simulink model "gm_sampleModel2016_3_sub"  (R2023a)
settings: Solver=VariableStepAuto  StartTime=0.0  StopTime=10.0  RelTol=1e-3
libraries: simulink x2
settings Model: Creator=user1  LastModifiedBy=user1
settings OptimizationCC: BlockReduction=off  ConditionallyExecuteInputs=off
settings DebuggingCC: InheritedTsInSrcMsg=none

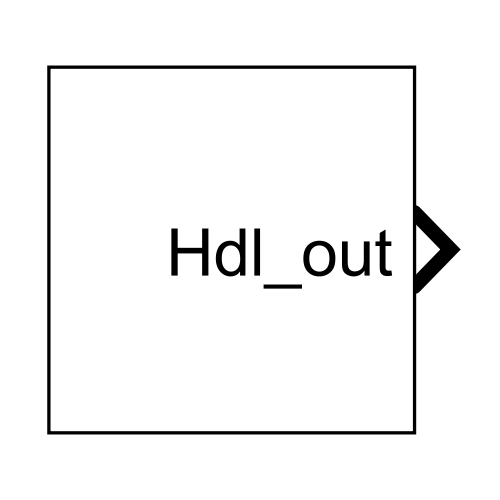
[thumbnail: Simulink's stored preview of the top-level diagram]
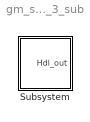
== system gm_sampleModel2016_3_sub ==
  Subsystem : Subsystem

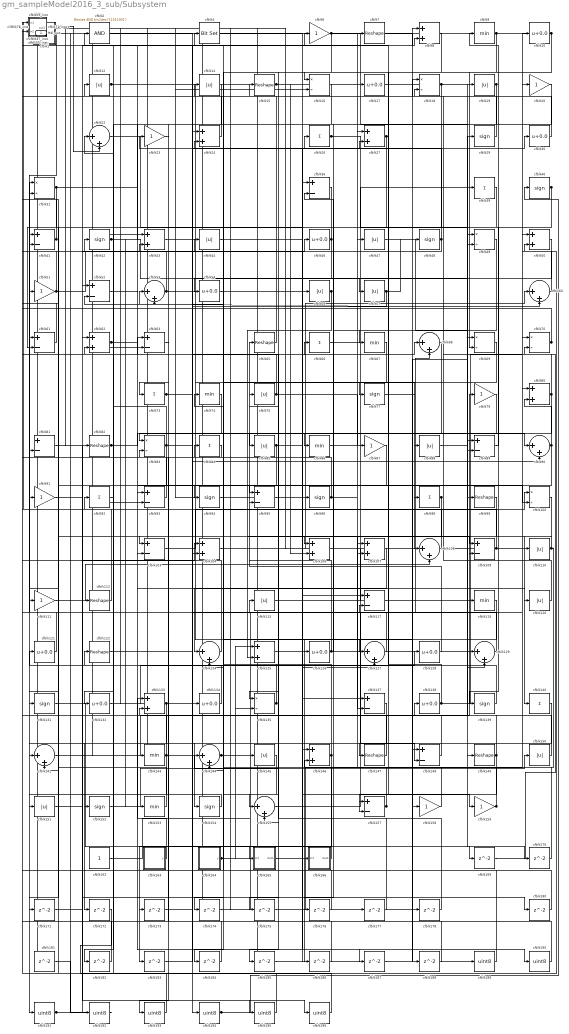
== system gm_sampleModel2016_3_sub/Subsystem ==
  cfblk1 : Subsystem  mask(Compare To Zero){relop=<=, OutDataTypeStr=uint8, ZeroCross=on}
      mask prompts: relop "Simulink:masks:Operator_MP"; OutDataTypeStr "Simulink:masks:OutputDataType_MP"; ZeroCross "Simulink:masks:EnableZerocrossingDetection_MP"
      mask help: Simulink:masks:CompareToZero_MD
      mask init:
      | OutDataTypeStr = 'uint8';
      | ZeroCross = 'on';
      | blkName = 'sampleModel2016_3_sub/Subsystem/cfblk1';
      | relop = '<=';
      | setValue = 'fixdt(0, 8)';
      mask TypeOptions relop: == | ~= | < | <= | >= | >
      mask TypeOptions OutDataTypeStr: Simulink:masks:uint8 | Simulink:masks:boolean
      mask Callback ZeroCross: sl('zeroCrossEnable', gcbh);
      mask Display: disp([relop,' 0'])
  cfblk{10,17,30,46,54,121,126,128,132,134,138} (11 alike) : Bias  Bias=0.0  SaturateOnIntegerOverflow=off
  cfblk{16,18,31,49,69..70,83,100,135} (9 alike) : Product  Inputs=*/  OutDataTypeStr=uint8  RndMeth=Zero  SaturateOnIntegerOverflow=on
  cfblk{36,41,52,61,63,81,89,93,95,103,109,117,137,148,157} (15 alike) : Sum  Inputs=+-  OutDataTypeStr=uint8
  cfblk{8,24,27,43,50,62,80,104,106..107,125,133,146} (13 alike) : Sum  OutDataTypeStr=uint8
  cfblk{22,53,60,68,90,108,124,127,129,141,144,155} (12 alike) : Sum  Inputs=|++  OutDataTypeStr=uint8
  cfblk{12,14,19,44,47,56..57,75,85,88,110,115,120,145,150..151} (16 alike) : Abs  OutDataTypeStr=uint8  SaturateOnIntegerOverflow=off
  cfblk{6,20,23,51,79,87,91,111,158..159} (10 alike) : Gain  OutDataTypeStr=uint8
  cfblk{7,15,65,82,99,112,122,147,149} (9 alike) : Reshape
  cfblk113_inst : Subsystem
  cfblk{9,67,74,86,119,143,153} (7 alike) : MinMax  OutDataTypeStr=uint8
  cfblk123_inst : Subsystem
  cfblk130_inst : Subsystem
  cfblk{29,40,42,48,77,94,96,131,139,152,154} (11 alike) : Signum
  cfblk13_inst : Subsystem
  cfblk{26,39,66,73,84,92,98,140} (8 alike) : Sum  Inputs=+  OutDataTypeStr=uint8
  cfblk156_inst : Subsystem
  cfblk162 : Constant  OutDataTypeStr=uint8  SampleTime=-1
  cfblk163 : Subsystem  mask(Counter Free-Running){NumBits=double(16), tsamp=double(-1)}
      mask prompts: NumBits "Simulink:masks:NumberOfBits_MP"; tsamp "Simulink:masks:SampleTime_MP"
      mask help: Simulink:masks:CounterFreeRunning_MD
  cfblk164 : Subsystem  mask(Counter Limited){uplimit=double(7), tsamp=double(-1)}
      mask prompts: uplimit "Simulink:masks:UpperLimit_MP"; tsamp "Simulink:masks:SampleTime_MP"
      mask help: Simulink:masks:CounterLimited_MD
      mask init:
      | nbits = double(8);
      | tsamp = double(-1);
      | uplimit = double(7);
  cfblk165 : Subsystem
  cfblk166 : Subsystem
  cfblk{169..178,180..188} (19 alike) : Delay  SampleTime=1
  cfblk{189..196} (8 alike) : DataTypeConversion  OutDataTypeStr=uint8  SaturateOnIntegerOverflow=off  RndMeth=Floor
  cfblk2 : simulink/Logic and Bit Operations/Bitwise Operator  logicop=AND  UseBitMask=on  BitMask=bin2dec('11011001')  BitMaskRealWorld=Stored Integer
      settings: LibrarySourceBlock=|
      | hdlsllib/Logic and Bit
      | Operations/Bitwise
      | Operator
  cfblk25_inst : Subsystem
  cfblk3 : Constant  Value=0  OutDataTypeStr=uint8  SampleTime=1
  cfblk37_inst : Subsystem
  cfblk4 : simulink/Logic and Bit Operations/Bit Set  iBit=0
      settings: LibrarySourceBlock=|
      | hdlsllib/Logic and Bit
      | Operations/Bit Set
  cfblk55_inst : Subsystem
  cfblk59_inst : Subsystem
  cfblk71_inst : Subsystem
  cfblk78_inst : Subsystem
  Hdl_out : Outport  OutDataTypeStr=uint8  SampleTime=1
  wires:
  cfblk1/1(y) -> cfblk191/1
  cfblk10/1 -> cfblk69/2, Hdl_out/1
  cfblk100/1 -> cfblk140/1
  cfblk103/1 -> cfblk100/1
  cfblk104/1 -> cfblk60/1
  cfblk106/1 -> cfblk148/2
  cfblk107/1 -> cfblk124/1
  cfblk108/1 -> cfblk37_inst/1(in1)
  cfblk109/1 -> cfblk78_inst/2(in2), cfblk31/1
  cfblk110/1 -> cfblk133/2, cfblk106/1
  cfblk111/1 -> cfblk108/2
  cfblk112/1 -> cfblk13_inst/1(in1)
  cfblk113_inst/1(out1) -> cfblk43/1
  cfblk115/1 -> cfblk39/1
  cfblk117/1 -> cfblk10/1
  cfblk119/1 -> cfblk184/1
  cfblk12/1 -> cfblk90/1, cfblk188/1
  cfblk120/1 -> cfblk18/2
  cfblk121/1 -> cfblk78_inst/1(in1)
  cfblk122/1 -> cfblk66/1
  cfblk123_inst/1(out1) -> cfblk19/1, cfblk134/1, cfblk16/2
  cfblk124/1 -> cfblk123_inst/1(in1)
  cfblk125/1 -> cfblk186/1
  cfblk126/1 -> cfblk65/1, cfblk36/2
  cfblk127/1 -> cfblk115/1
  cfblk128/1 -> cfblk95/2
  cfblk129/1 -> cfblk61/1
  cfblk13_inst/1(out1) -> cfblk189/1
  cfblk130_inst/1(out1) -> cfblk110/1
  cfblk131/1 -> cfblk169/1
  cfblk132/1 -> cfblk128/1
  cfblk133/1 -> cfblk68/1, cfblk141/2
  cfblk134/1 -> cfblk121/1
  cfblk135/1 -> cfblk52/2, cfblk84/1
  cfblk137/1 -> cfblk172/1
  cfblk138/1 -> cfblk130_inst/2(in2), cfblk20/1
  cfblk139/1 -> cfblk122/1
  cfblk14/1 -> cfblk182/1
  cfblk140/1 -> cfblk154/1
  cfblk141/1 -> cfblk49/2
  cfblk143/1 -> cfblk55_inst/2(in2), cfblk151/1
  cfblk144/1 -> cfblk70/1, cfblk135/2
  cfblk145/1 -> cfblk174/1
  cfblk146/1 -> cfblk24/2, cfblk183/1
  cfblk147/1 -> cfblk74/1
  cfblk148/1 -> cfblk75/1
  cfblk149/1 -> cfblk157/2, cfblk79/1
  cfblk15/1 -> cfblk146/1, cfblk117/1, cfblk106/2
  cfblk150/1 -> cfblk12/1
  cfblk151/1 -> cfblk112/1
  cfblk152/1 -> cfblk150/1
  cfblk153/1 -> cfblk51/1
  cfblk154/1 -> cfblk152/1
  cfblk155/1 -> cfblk68/2
  cfblk156_inst/1(out1) -> cfblk63/2, cfblk143/1
  cfblk157/1 -> cfblk62/2, cfblk53/1
  cfblk158/1 -> cfblk92/1
  cfblk159/1 -> cfblk146/2, cfblk14/1
  cfblk16/1 -> cfblk103/1
  cfblk162/1 -> cfblk109/2
  cfblk163/1(y) -> cfblk133/1
  cfblk164/1(y) -> cfblk138/1, cfblk125/1
  cfblk165/1(Out1) -> cfblk47/1
  cfblk166/1(Out1) -> cfblk36/1
  cfblk169/1 -> cfblk70/2
  cfblk17/1 -> cfblk157/1
  cfblk170/1 -> cfblk124/2
  cfblk171/1 -> cfblk104/1
  cfblk172/1 -> cfblk50/2
  cfblk173/1 -> cfblk60/2
  cfblk174/1 -> cfblk107/1
  cfblk175/1 -> cfblk80/1
  cfblk176/1 -> cfblk156_inst/2(in2)
  cfblk177/1 -> cfblk144/1
  cfblk178/1 -> cfblk63/1
  cfblk18/1 -> cfblk131/1, cfblk170/1
  cfblk180/1 -> cfblk25_inst/2(in2)
  cfblk181/1 -> cfblk192/1
  cfblk182/1 -> cfblk123_inst/2(in2)
  cfblk183/1 -> cfblk117/2
  cfblk184/1 -> cfblk71_inst/2(in2)
  cfblk185/1 -> cfblk127/2
  cfblk186/1 -> cfblk24/1
  cfblk187/1 -> cfblk69/1
  cfblk188/1 -> cfblk83/2
  cfblk189/1 -> cfblk4/1
  cfblk19/1 -> cfblk135/1, cfblk86/1
  cfblk190/1 -> cfblk148/1
  cfblk191/1 -> cfblk46/1, cfblk6/1
  cfblk192/1 -> cfblk1/1(u)
  cfblk193/1 -> cfblk2/1
  cfblk194/1 -> cfblk40/1, cfblk196/1
  cfblk195/1 -> cfblk130_inst/1(in1)
  cfblk196/1 -> cfblk91/1
  cfblk2/1 -> cfblk194/1
  cfblk20/1 -> cfblk103/2
  cfblk22/1 -> cfblk166/1(In1)
  cfblk23/1 -> cfblk73/1
  cfblk24/1 -> cfblk71_inst/1(in1)
  cfblk25_inst/1(out1) -> cfblk96/1, cfblk82/1
  cfblk26/1 -> cfblk89/1, cfblk129/2
  cfblk27/1 -> cfblk61/2, cfblk57/1
  cfblk29/1 -> cfblk59_inst/1(in1)
  cfblk3/1 -> cfblk22/2, cfblk181/1
  cfblk30/1 -> cfblk18/1
  cfblk31/1 -> cfblk93/1, cfblk41/2
  cfblk36/1 -> cfblk85/1
  cfblk37_inst/1(out1) -> cfblk56/1
  cfblk39/1 -> cfblk147/1
  cfblk4/1 -> cfblk190/1
  cfblk40/1 -> cfblk155/2, cfblk139/1
  cfblk41/1 -> cfblk55_inst/1(in1), cfblk113_inst/2(in2)
  cfblk42/1 -> cfblk99/1, cfblk8/2, cfblk153/1
  cfblk43/1 -> cfblk77/1
  cfblk44/1 -> cfblk27/2
  cfblk46/1 -> cfblk41/1, cfblk165/1(In1)
  cfblk47/1 -> cfblk149/1
  cfblk48/1 -> cfblk43/2, cfblk23/1
  cfblk49/1 -> cfblk176/1
  cfblk50/1 -> cfblk144/2
  cfblk51/1 -> cfblk44/1, cfblk37_inst/2(in2)
  cfblk52/1 -> cfblk187/1
  cfblk53/1 -> cfblk59_inst/2(in2), cfblk108/1
  cfblk54/1 -> cfblk137/1
  cfblk55_inst/1(out1) -> cfblk81/1, cfblk145/1
  cfblk56/1 -> cfblk125/2, cfblk185/1
  cfblk57/1 -> cfblk53/2, cfblk48/1
  cfblk59_inst/1(out1) -> cfblk178/1, cfblk177/1
  cfblk6/1 -> cfblk89/2, cfblk16/1
  cfblk60/1 -> cfblk50/1
  cfblk61/1 -> cfblk25_inst/1(in1)
  cfblk62/1 -> cfblk120/1, cfblk180/1
  cfblk63/1 -> cfblk193/1
  cfblk65/1 -> cfblk15/1
  cfblk66/1 -> cfblk29/1
  cfblk67/1 -> cfblk126/1
  cfblk68/1 -> cfblk175/1
  cfblk69/1 -> cfblk94/1
  cfblk7/1 -> cfblk158/1
  cfblk70/1 -> cfblk156_inst/1(in1), cfblk31/2
  cfblk71_inst/1(out1) -> cfblk93/2, cfblk17/1, cfblk119/1
  cfblk73/1 -> cfblk8/1, cfblk26/1
  cfblk74/1 -> cfblk83/1
  cfblk75/1 -> cfblk113_inst/1(in1), cfblk87/1
  cfblk77/1 -> cfblk98/1
  cfblk78_inst/1(out1) -> cfblk129/1
  cfblk79/1 -> cfblk127/1
  cfblk8/1 -> cfblk54/1
  cfblk80/1 -> cfblk52/1, cfblk104/2
  cfblk81/1 -> cfblk173/1
  cfblk82/1 -> cfblk88/1, cfblk100/2
  cfblk83/1 -> cfblk90/2, cfblk42/1, cfblk132/1
  cfblk84/1 -> cfblk81/2
  cfblk85/1 -> cfblk141/1, cfblk159/1
  cfblk86/1 -> cfblk27/1
  cfblk87/1 -> cfblk95/1
  cfblk88/1 -> cfblk49/1
  cfblk89/1 -> cfblk9/1
  cfblk9/1 -> cfblk155/1, cfblk67/1
  cfblk90/1 -> cfblk80/2, cfblk111/1
  cfblk91/1 -> cfblk195/1
  cfblk92/1 -> cfblk22/1
  cfblk93/1 -> cfblk62/1
  cfblk94/1 -> cfblk109/1
  cfblk95/1 -> cfblk30/1
  cfblk96/1 -> cfblk7/1, cfblk13_inst/2(in2)
  cfblk98/1 -> cfblk137/2, cfblk171/1
  cfblk99/1 -> cfblk107/2

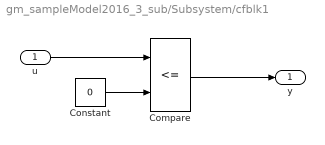
== system gm_sampleModel2016_3_sub/Subsystem/cfblk1 ==
  u : Inport  OutDataTypeStr=uint8  SampleTime=1
  Compare : RelationalOperator  Operator=<=  OutDataTypeStr=fixdt(0, 8)
  Constant : Constant  DisableCoverage=on  Value=0  OutDataTypeStr=Inherit: Inherit via back propagation  SampleTime=-1  PreserveConstantTs=on
  y : Outport  SampleTime=1
  wires:
  u/1 -> Compare/1
  Compare/1 -> y/1
  Constant/1 -> Compare/2

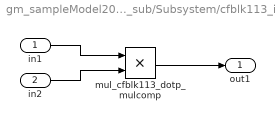
== system gm_sampleModel2016_3_sub/Subsystem/cfblk113_inst ==
  in1 : Inport  OutDataTypeStr=uint8  SampleTime=1
  in2 : Inport  Port=2  OutDataTypeStr=uint8  SampleTime=1
  mul_cfblk113_dotp_mulcomp : Product  Inputs=**  OutDataTypeStr=uint8  SampleTime=1
  out1 : Outport  OutDataTypeStr=uint8  SampleTime=1
  wires:
  in1/1 -> mul_cfblk113_dotp_mulcomp/1
  in2/1 -> mul_cfblk113_dotp_mulcomp/2
  mul_cfblk113_dotp_mulcomp/1 -> out1/1

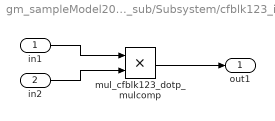
== system gm_sampleModel2016_3_sub/Subsystem/cfblk123_inst ==
  in1 : Inport  OutDataTypeStr=uint8  SampleTime=1
  in2 : Inport  Port=2  OutDataTypeStr=uint8  SampleTime=1
  mul_cfblk123_dotp_mulcomp : Product  Inputs=**  OutDataTypeStr=uint8  SampleTime=1
  out1 : Outport  OutDataTypeStr=uint8  SampleTime=1
  wires:
  in1/1 -> mul_cfblk123_dotp_mulcomp/1
  in2/1 -> mul_cfblk123_dotp_mulcomp/2
  mul_cfblk123_dotp_mulcomp/1 -> out1/1

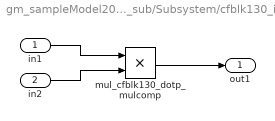
== system gm_sampleModel2016_3_sub/Subsystem/cfblk130_inst ==
  in1 : Inport  OutDataTypeStr=uint8  SampleTime=1
  in2 : Inport  Port=2  OutDataTypeStr=uint8  SampleTime=1
  mul_cfblk130_dotp_mulcomp : Product  Inputs=**  OutDataTypeStr=uint8  SampleTime=1
  out1 : Outport  OutDataTypeStr=uint8  SampleTime=1
  wires:
  in1/1 -> mul_cfblk130_dotp_mulcomp/1
  in2/1 -> mul_cfblk130_dotp_mulcomp/2
  mul_cfblk130_dotp_mulcomp/1 -> out1/1

== system gm_sampleModel2016_3_sub/Subsystem/cfblk13_inst ==
  in1 : Inport  OutDataTypeStr=uint8  SampleTime=1
  in2 : Inport  Port=2  OutDataTypeStr=uint8  SampleTime=1
  mul_cfblk13_dotp_mulcomp : Product  Inputs=**  OutDataTypeStr=uint8  SampleTime=1
  out1 : Outport  OutDataTypeStr=uint8  SampleTime=1
  wires:
  in1/1 -> mul_cfblk13_dotp_mulcomp/1
  in2/1 -> mul_cfblk13_dotp_mulcomp/2
  mul_cfblk13_dotp_mulcomp/1 -> out1/1

== system gm_sampleModel2016_3_sub/Subsystem/cfblk156_inst ==
  in1 : Inport  OutDataTypeStr=uint8  SampleTime=1
  in2 : Inport  Port=2  OutDataTypeStr=uint8  SampleTime=1
  mul_cfblk156_dotp_mulcomp : Product  Inputs=**  OutDataTypeStr=uint8  SampleTime=1
  out1 : Outport  OutDataTypeStr=uint8  SampleTime=1
  wires:
  in1/1 -> mul_cfblk156_dotp_mulcomp/1
  in2/1 -> mul_cfblk156_dotp_mulcomp/2
  mul_cfblk156_dotp_mulcomp/1 -> out1/1

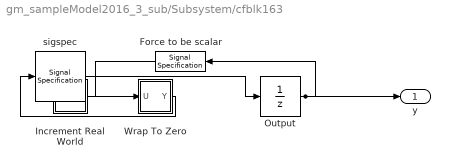
== system gm_sampleModel2016_3_sub/Subsystem/cfblk163 ==
  Force to be scalar : SignalSpecification  DisableCoverage=on  Dimensions=1
  Increment Real World : Subsystem  mask(Real World Value Increment){}
      mask help: Simulink:masks:RealWorldValueIncrement_MD
      mask Display: disp('V++')
  Output : UnitDelay  InitialCondition=0.0  SampleTime=tsamp  HasFrameUpgradeWarning=on
  Wrap To Zero : Subsystem  mask(Wrap To Zero){Threshold=double(65535)}
      mask prompts: Threshold "Simulink:masks:Threshold_MP"
      mask help: Simulink:masks:WrapToZero_MD
  sigspec : SignalSpecification  OutDataTypeStr=uint16  Dimensions=1
  y : Outport  SampleTime=1
  wires:
  Force to be scalar/1 -> Increment Real World/1(u)
  Increment Real World/1(y) -> Wrap To Zero/1(U)
  Output/1 -> Force to be scalar/1, y/1
  Wrap To Zero/1(Y) -> sigspec/1
  sigspec/1 -> Output/1

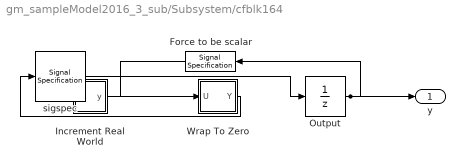
== system gm_sampleModel2016_3_sub/Subsystem/cfblk164 ==
  Force to be scalar : SignalSpecification  DisableCoverage=on  Dimensions=1
  Increment Real World : Subsystem  mask(Real World Value Increment){}
      mask help: Simulink:masks:RealWorldValueIncrement_MD
      mask Display: disp('V++')
  Output : UnitDelay  InitialCondition=0.0  SampleTime=tsamp  HasFrameUpgradeWarning=on
  Wrap To Zero : Subsystem  mask(Wrap To Zero){Threshold=double(7)}
      mask prompts: Threshold "Simulink:masks:Threshold_MP"
      mask help: Simulink:masks:WrapToZero_MD
  sigspec : SignalSpecification  OutDataTypeStr=uint8  Dimensions=1
  y : Outport  SampleTime=1
  wires:
  Force to be scalar/1 -> Increment Real World/1(u)
  Increment Real World/1(y) -> Wrap To Zero/1(U)
  Output/1 -> Force to be scalar/1, y/1
  Wrap To Zero/1(Y) -> sigspec/1
  sigspec/1 -> Output/1

== system gm_sampleModel2016_3_sub/Subsystem/cfblk165 ==
  In1 : Inport  OutDataTypeStr=uint8  PortDimensions=1  SampleTime=1
  Out1 : Outport  SampleTime=1
  wires:
  In1/1 -> Out1/1

== system gm_sampleModel2016_3_sub/Subsystem/cfblk166 ==
  In1 : Inport  OutDataTypeStr=uint8  PortDimensions=1  SampleTime=1
  Out1 : Outport  SampleTime=1
  wires:
  In1/1 -> Out1/1

== system gm_sampleModel2016_3_sub/Subsystem/cfblk25_inst ==
  in1 : Inport  OutDataTypeStr=uint8  SampleTime=1
  in2 : Inport  Port=2  OutDataTypeStr=uint8  SampleTime=1
  mul_cfblk25_dotp_mulcomp : Product  Inputs=**  OutDataTypeStr=uint8  SampleTime=1
  out1 : Outport  OutDataTypeStr=uint8  SampleTime=1
  wires:
  in1/1 -> mul_cfblk25_dotp_mulcomp/1
  in2/1 -> mul_cfblk25_dotp_mulcomp/2
  mul_cfblk25_dotp_mulcomp/1 -> out1/1

== system gm_sampleModel2016_3_sub/Subsystem/cfblk37_inst ==
  in1 : Inport  OutDataTypeStr=uint8  SampleTime=1
  in2 : Inport  Port=2  OutDataTypeStr=uint8  SampleTime=1
  mul_cfblk37_dotp_mulcomp : Product  Inputs=**  OutDataTypeStr=uint8  SampleTime=1
  out1 : Outport  OutDataTypeStr=uint8  SampleTime=1
  wires:
  in1/1 -> mul_cfblk37_dotp_mulcomp/1
  in2/1 -> mul_cfblk37_dotp_mulcomp/2
  mul_cfblk37_dotp_mulcomp/1 -> out1/1

== system gm_sampleModel2016_3_sub/Subsystem/cfblk55_inst ==
  in1 : Inport  OutDataTypeStr=uint8  SampleTime=1
  in2 : Inport  Port=2  OutDataTypeStr=uint8  SampleTime=1
  mul_cfblk55_dotp_mulcomp : Product  Inputs=**  OutDataTypeStr=uint8  SampleTime=1
  out1 : Outport  OutDataTypeStr=uint8  SampleTime=1
  wires:
  in1/1 -> mul_cfblk55_dotp_mulcomp/1
  in2/1 -> mul_cfblk55_dotp_mulcomp/2
  mul_cfblk55_dotp_mulcomp/1 -> out1/1

== system gm_sampleModel2016_3_sub/Subsystem/cfblk59_inst ==
  in1 : Inport  OutDataTypeStr=uint8  SampleTime=1
  in2 : Inport  Port=2  OutDataTypeStr=uint8  SampleTime=1
  mul_cfblk59_dotp_mulcomp : Product  Inputs=**  OutDataTypeStr=uint8  SampleTime=1
  out1 : Outport  OutDataTypeStr=uint8  SampleTime=1
  wires:
  in1/1 -> mul_cfblk59_dotp_mulcomp/1
  in2/1 -> mul_cfblk59_dotp_mulcomp/2
  mul_cfblk59_dotp_mulcomp/1 -> out1/1

== system gm_sampleModel2016_3_sub/Subsystem/cfblk71_inst ==
  in1 : Inport  OutDataTypeStr=uint8  SampleTime=1
  in2 : Inport  Port=2  OutDataTypeStr=uint8  SampleTime=1
  mul_cfblk71_dotp_mulcomp : Product  Inputs=**  OutDataTypeStr=uint8  SampleTime=1
  out1 : Outport  OutDataTypeStr=uint8  SampleTime=1
  wires:
  in1/1 -> mul_cfblk71_dotp_mulcomp/1
  in2/1 -> mul_cfblk71_dotp_mulcomp/2
  mul_cfblk71_dotp_mulcomp/1 -> out1/1

== system gm_sampleModel2016_3_sub/Subsystem/cfblk78_inst ==
  in1 : Inport  OutDataTypeStr=uint8  SampleTime=1
  in2 : Inport  Port=2  OutDataTypeStr=uint8  SampleTime=1
  mul_cfblk78_dotp_mulcomp : Product  Inputs=**  OutDataTypeStr=uint8  SampleTime=1
  out1 : Outport  OutDataTypeStr=uint8  SampleTime=1
  wires:
  in1/1 -> mul_cfblk78_dotp_mulcomp/1
  in2/1 -> mul_cfblk78_dotp_mulcomp/2
  mul_cfblk78_dotp_mulcomp/1 -> out1/1

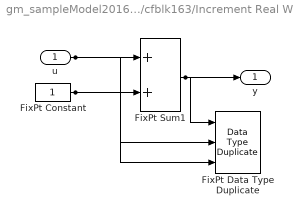
== system gm_sampleModel2016_3_sub/Subsystem/cfblk163/Increment Real World ==
  u : Inport  OutDataTypeStr=uint16  SampleTime=1
  FixPt Constant : Constant  DisableCoverage=on  OutDataTypeStr=Inherit: Inherit via back propagation  SampleTime=-1
  FixPt Data Type Duplicate : DataTypeDuplicate  DisableCoverage=on  NumInputPorts=3
  FixPt Sum1 : Sum  InputSameDT=on  OutDataTypeStr=Inherit: Inherit via back propagation  LockScale=on
  y : Outport  SampleTime=1
  wires:
  u/1 -> FixPt Sum1/1, FixPt Data Type Duplicate/2
  FixPt Constant/1 -> FixPt Sum1/2, FixPt Data Type Duplicate/3
  FixPt Sum1/1 -> FixPt Data Type Duplicate/1, y/1

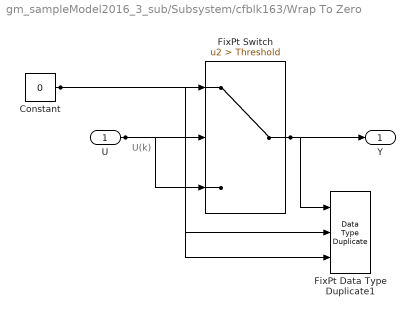
== system gm_sampleModel2016_3_sub/Subsystem/cfblk163/Wrap To Zero ==
  note: U(k)
  U : Inport  OutDataTypeStr=uint16  SampleTime=1
  Constant : Constant  DisableCoverage=on  Value=0  OutDataTypeStr=Inherit: Inherit via back propagation  SampleTime=-1
  FixPt Data Type Duplicate1 : DataTypeDuplicate  DisableCoverage=on  NumInputPorts=3
  FixPt Switch : Switch  Criteria=u2 > Threshold  Threshold=Threshold  OutDataTypeStr=Inherit: Inherit via back propagation  ZeroCross=off  SaturateOnIntegerOverflow=off  InputSameDT=off
  Y : Outport  SampleTime=1
  wires:
  U/1 -> FixPt Switch/3, FixPt Switch/2, FixPt Data Type Duplicate1/2
  Constant/1 -> FixPt Switch/1, FixPt Data Type Duplicate1/3
  FixPt Switch/1 -> FixPt Data Type Duplicate1/1, Y/1

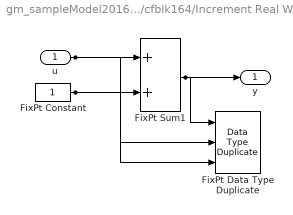
== system gm_sampleModel2016_3_sub/Subsystem/cfblk164/Increment Real World ==
  u : Inport  OutDataTypeStr=uint8  SampleTime=1
  FixPt Constant : Constant  DisableCoverage=on  OutDataTypeStr=Inherit: Inherit via back propagation  SampleTime=-1
  FixPt Data Type Duplicate : DataTypeDuplicate  DisableCoverage=on  NumInputPorts=3
  FixPt Sum1 : Sum  InputSameDT=on  OutDataTypeStr=Inherit: Inherit via back propagation  LockScale=on
  y : Outport  SampleTime=1
  wires:
  u/1 -> FixPt Sum1/1, FixPt Data Type Duplicate/2
  FixPt Constant/1 -> FixPt Sum1/2, FixPt Data Type Duplicate/3
  FixPt Sum1/1 -> FixPt Data Type Duplicate/1, y/1

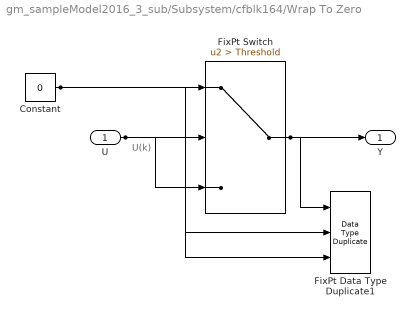
== system gm_sampleModel2016_3_sub/Subsystem/cfblk164/Wrap To Zero ==
  note: U(k)
  U : Inport  OutDataTypeStr=uint8  SampleTime=1
  Constant : Constant  DisableCoverage=on  Value=0  OutDataTypeStr=Inherit: Inherit via back propagation  SampleTime=-1
  FixPt Data Type Duplicate1 : DataTypeDuplicate  DisableCoverage=on  NumInputPorts=3
  FixPt Switch : Switch  Criteria=u2 > Threshold  Threshold=Threshold  OutDataTypeStr=Inherit: Inherit via back propagation  ZeroCross=off  SaturateOnIntegerOverflow=off  InputSameDT=off
  Y : Outport  SampleTime=1
  wires:
  U/1 -> FixPt Switch/3, FixPt Switch/2, FixPt Data Type Duplicate1/2
  Constant/1 -> FixPt Switch/1, FixPt Data Type Duplicate1/3
  FixPt Switch/1 -> FixPt Data Type Duplicate1/1, Y/1
